simulink model "sofc_system5_mpc11_int"  (Simulink 7.6)
settings: Solver=FixedStepDiscrete  StartTime=0.0  StopTime=3500  FixedStep=1  MaxStep=1  RelTol=1e-3
settings Model: Creator=Ben  LastModifiedBy=Ben

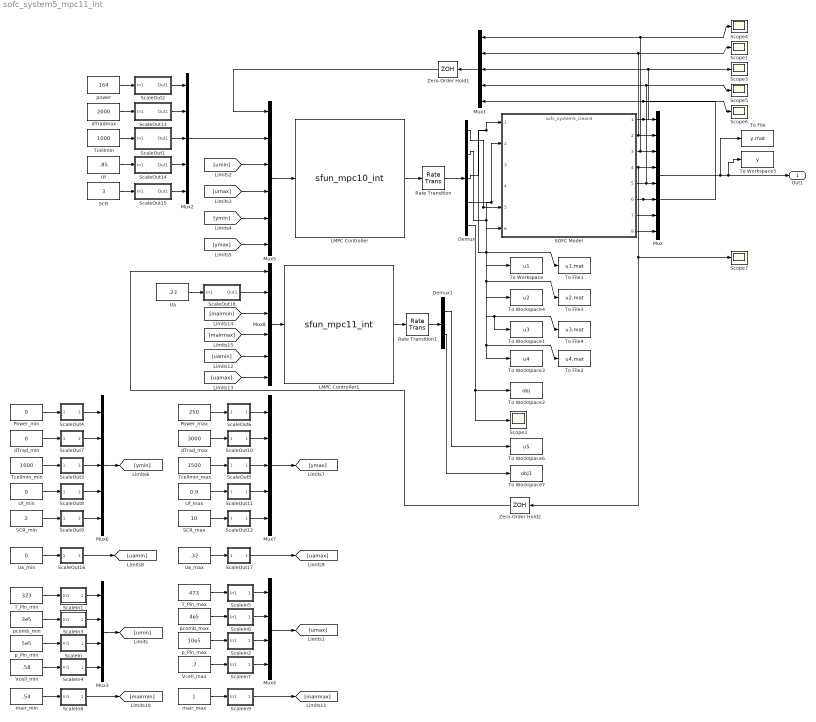
== system sofc_system5_mpc11_int ==
  Demux : Demux  Outputs=5
  Demux1 : Demux  Outputs=2
  LMPC Controller : S-Function  Priority=3  FunctionName=sfun_mpc10_int  EnableBusSupport=off
  LMPC Controller1 : S-Function  Priority=3  FunctionName=sfun_mpc11_int  EnableBusSupport=off
  Mux : Mux  Inputs=8
  Mux{1..2,6..7} (4 alike) : Mux  Inputs=5
  Mux3 : Mux
  Mux4 : Mux
  Mux5 : Mux  Inputs=6
  Mux8 : Mux  Inputs=6
  Power_max : Constant  Priority=1  Value=250
  Power_min : Constant  Priority=1  Value=0
  Rate Transition : RateTransition  Deterministic=off  OutPortSampleTimeMultiple=5  OutPortSampleTime=1
  Rate Transition1 : RateTransition  Deterministic=off  OutPortSampleTimeMultiple=5  OutPortSampleTime=1
  SCR : Constant  Priority=1  Value=3
  SCR_max : Constant  Priority=1  Value=10
  SCR_min : Constant  Priority=1  Value=2
  SOFC Model : ModelReference  Priority=1  ModelNameDialog=sofc_system5_clean3  SimulationMode=Normal  ModelReferenceVersion=1.62  CopyOfModelName=sofc_system5_clean3
      mask Display: image(imread('sofc.png'))
  ScaleIn : Subsystem
  ScaleIn1 : Subsystem
  ScaleIn2 : Subsystem
  ScaleIn3 : Subsystem
  ScaleIn4 : Subsystem
  ScaleIn5 : Subsystem
  ScaleIn6 : Subsystem
  ScaleIn7 : Subsystem
  ScaleIn8 : Subsystem
  ScaleIn9 : Subsystem
  ScaleOut1 : Subsystem  Priority=1
  ScaleOut10 : Subsystem  Priority=1
  ScaleOut11 : Subsystem  Priority=1
  ScaleOut12 : Subsystem  Priority=1
  ScaleOut13 : Subsystem  Priority=1
  ScaleOut14 : Subsystem  Priority=1
  ScaleOut15 : Subsystem  Priority=1
  ScaleOut16 : Subsystem  Priority=1
  ScaleOut17 : Subsystem  Priority=1
  ScaleOut18 : Subsystem  Priority=1
  ScaleOut2 : Subsystem  Priority=1
  ScaleOut3 : Subsystem  Priority=1
  ScaleOut4 : Subsystem  Priority=1
  ScaleOut5 : Subsystem  Priority=1
  ScaleOut6 : Subsystem  Priority=1
  ScaleOut7 : Subsystem  Priority=1
  ScaleOut8 : Subsystem  Priority=1
  ScaleOut9 : Subsystem  Priority=1
  Scope{1..7} (7 alike) : Scope
      Scope1 settings: YMin=-0.125  YMax=0.15
      Scope2 settings: TimeRange=43.34600760456274  YMin=1645  YMax=1670  SaveName=ScopeData2
      Scope3 settings: YMin=1.85446  YMax=2.04966
      Scope4 settings: YMin=1.4787  YMax=1.4799  SaveName=ScopeData4
      Scope5 settings: YMin=-0.125  YMax=0.15  SaveName=ScopeData3
      Scope6 settings: YMin=-0.125  YMax=0.15  SaveName=ScopeData5
      Scope7 settings: YMin=-0.125  YMax=0.15  SaveName=ScopeData6
  T_Pin_max : Constant  Priority=1  Value=473
  T_Pin_min : Constant  Priority=1  Value=323
  Tcellmin : Constant  Priority=1  Value=1000
  Tcellmin_max : Constant  Priority=1  Value=1500
  Tcellmin_min : Constant  Priority=1  Value=1000
  To File : ToFile  Filename=y.mat
  To File1 : ToFile  Filename=u1.mat
  To File2 : ToFile  Filename=u4.mat
  To File3 : ToFile  Filename=u2.mat
  To File4 : ToFile  Filename=u3.mat
  To Workspace : ToWorkspace  VariableName=u1  SampleTime=-1  SaveFormat=Structure
  To Workspace1 : ToWorkspace  VariableName=u3  SampleTime=-1  SaveFormat=Structure
  To Workspace2 : ToWorkspace  VariableName=obj  SampleTime=-1  SaveFormat=Structure
  To Workspace3 : ToWorkspace  VariableName=u4  SampleTime=-1  SaveFormat=Structure
  To Workspace4 : ToWorkspace  VariableName=u2  SampleTime=-1  SaveFormat=Structure
  To Workspace5 : ToWorkspace  VariableName=y  SampleTime=-1  SaveFormat=Structure
  To Workspace6 : ToWorkspace  VariableName=u5  SampleTime=-1  SaveFormat=Structure
  To Workspace7 : ToWorkspace  VariableName=obj1  SampleTime=-1  SaveFormat=Structure
  Ua : Constant  Priority=1  Value=.23
  Ua_max : Constant  Priority=1  Value=.32
  Ua_min : Constant  Priority=1  Value=0
  Uf : Constant  Priority=1  Value=.85
  Uf_max : Constant  Priority=1  Value=0.9
  Uf_min : Constant  Priority=1  Value=0
  Vcell_max : Constant  Priority=1  Value=.7
  Vcell_min : Constant  Priority=1  Value=.58
  Zero-Order Hold1 : ZeroOrderHold  SampleTime=10
  Zero-Order Hold2 : ZeroOrderHold  SampleTime=10
  dTrad_max : Constant  Priority=1  Value=3000
  dTrad_min : Constant  Priority=1  Value=0
  dTradmax : Constant  Priority=1  Value=2000
  mair_max : Constant  Priority=1
  mair_min : Constant  Priority=1  Value=.54
  p_Pin_max : Constant  Priority=1  Value=10e5
  p_Pin_min : Constant  Priority=1  Value=5e5
  pcomb_max : Constant  Priority=1  Value=4e5
  pcomb_min : Constant  Priority=1  Value=3e5
  power : Constant  Priority=1  Value=164
  Out1 : Outport
  wires:
  SOFC Model/1 -> Mux/1, Mux1/3, Scope3/1
  SOFC Model/2 -> Mux/2, Mux1/2, Scope1/1
  SOFC Model/3 -> Mux/3, Mux1/1, Scope4/1
  SOFC Model/4 -> Mux/4, Scope7/1, Zero-Order Hold2/1
  SOFC Model/5 -> Mux/5, Mux1/4, Scope5/1
  SOFC Model/6 -> Mux/6, Scope6/1, Mux1/5
  Mux/1 -> Out1/1, To Workspace5/1, To File/1
  p_Pin_min/1 -> ScaleIn/1(In1)
  [umin] -> Mux5/3
  [umax] -> Mux5/4
  Mux5/1 -> LMPC Controller/1
  Zero-Order Hold1/1 -> Mux5/1
  power/1 -> ScaleOut2/1(In1)
  ScaleOut2/1(Out1) -> Mux2/1
  Mux2/1 -> Mux5/2
  T_Pin_min/1 -> ScaleIn1/1(In1)
  Mux3/1 -> [umin]
  Mux1/1 -> Zero-Order Hold1/1
  [ymax] -> Mux5/6
  [ymin] -> Mux5/5
  Power_min/1 -> ScaleOut4/1(In1)
  Tcellmin_min/1 -> ScaleOut3/1(In1)
  Mux6/1 -> [ymin]
  ScaleOut4/1(Out1) -> Mux6/1
  SOFC Model/7 -> Mux/7
  SOFC Model/8 -> Mux/8
  LMPC Controller/1 -> Rate Transition/1
  Rate Transition/1 -> Demux/1
  Demux/5 -> Scope2/1, To Workspace2/1
  Tcellmin/1 -> ScaleOut1/1(In1)
  ScaleOut3/1(Out1) -> Mux6/3
  dTrad_min/1 -> ScaleOut7/1(In1)
  ScaleOut7/1(Out1) -> Mux6/2
  Uf_min/1 -> ScaleOut8/1(In1)
  ScaleOut8/1(Out1) -> Mux6/4
  SCR_min/1 -> ScaleOut9/1(In1)
  ScaleOut9/1(Out1) -> Mux6/5
  Power_max/1 -> ScaleOut6/1(In1)
  Tcellmin_max/1 -> ScaleOut5/1(In1)
  Mux7/1 -> [ymax]
  ScaleOut6/1(Out1) -> Mux7/1
  ScaleOut5/1(Out1) -> Mux7/3
  dTrad_max/1 -> ScaleOut10/1(In1)
  ScaleOut10/1(Out1) -> Mux7/2
  Uf_max/1 -> ScaleOut11/1(In1)
  ScaleOut11/1(Out1) -> Mux7/4
  SCR_max/1 -> ScaleOut12/1(In1)
  ScaleOut12/1(Out1) -> Mux7/5
  ScaleIn1/1(Out1) -> Mux3/1
  ScaleIn/1(Out1) -> Mux3/3
  pcomb_min/1 -> ScaleIn3/1(In1)
  ScaleIn3/1(Out1) -> Mux3/2
  Vcell_min/1 -> ScaleIn4/1(In1)
  ScaleIn4/1(Out1) -> Mux3/4
  p_Pin_max/1 -> ScaleIn2/1(In1)
  T_Pin_max/1 -> ScaleIn5/1(In1)
  Mux4/1 -> [umax]
  ScaleIn5/1(Out1) -> Mux4/1
  ScaleIn2/1(Out1) -> Mux4/3
  pcomb_max/1 -> ScaleIn6/1(In1)
  ScaleIn6/1(Out1) -> Mux4/2
  Vcell_max/1 -> ScaleIn7/1(In1)
  ScaleIn7/1(Out1) -> Mux4/4
  ScaleOut1/1(Out1) -> Mux2/3
  dTradmax/1 -> ScaleOut13/1(In1)
  ScaleOut13/1(Out1) -> Mux2/2
  Uf/1 -> ScaleOut14/1(In1)
  ScaleOut14/1(Out1) -> Mux2/4
  SCR/1 -> ScaleOut15/1(In1)
  ScaleOut15/1(Out1) -> Mux2/5
  Demux/3 -> SOFC Model/1, To Workspace/1, To File1/1
  Demux/4 -> SOFC Model/2, To Workspace4/1, To File3/1
  Demux/2 -> SOFC Model/6, To Workspace3/1, To File2/1
  Demux/1 -> SOFC Model/5, To Workspace1/1, To File4/1
  Ua_min/1 -> ScaleOut16/1(In1)
  ScaleOut16/1(Out1) -> [uamin]
  Ua_max/1 -> ScaleOut17/1(In1)
  ScaleOut17/1(Out1) -> [uamax]
  mair_min/1 -> ScaleIn8/1(In1)
  ScaleIn8/1(Out1) -> [mairmin]
  mair_max/1 -> ScaleIn9/1(In1)
  ScaleIn9/1(Out1) -> [mairmax]
  Ua/1 -> ScaleOut18/1(In1)
  ScaleOut18/1(Out1) -> Mux8/2
  [uamax] -> Mux8/6
  [uamin] -> Mux8/5
  [mairmax] -> Mux8/4
  [mairmin] -> Mux8/3
  Mux8/1 -> LMPC Controller1/1
  LMPC Controller1/1 -> Rate Transition1/1
  Zero-Order Hold2/1 -> Mux8/1
  Rate Transition1/1 -> Demux1/1
  Demux1/1 -> To Workspace6/1
  Demux1/2 -> To Workspace7/1

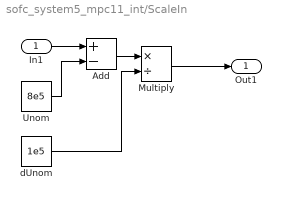
== system sofc_system5_mpc11_int/ScaleIn ==
  In1 : Inport
  Add : Sum  Inputs=+-
  Multiply : Product  Inputs=*/
  Unom : Constant  Value=8e5
  dUnom : Constant  Value=1e5
  Out1 : Outport
  wires:
  Unom/1 -> Add/2
  In1/1 -> Add/1
  Add/1 -> Multiply/1
  dUnom/1 -> Multiply/2
  Multiply/1 -> Out1/1

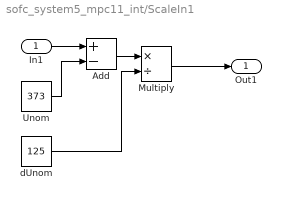
== system sofc_system5_mpc11_int/ScaleIn1 ==
  In1 : Inport
  Add : Sum  Inputs=+-
  Multiply : Product  Inputs=*/
  Unom : Constant  Value=373
  dUnom : Constant  Value=125
  Out1 : Outport
  wires:
  Unom/1 -> Add/2
  In1/1 -> Add/1
  Add/1 -> Multiply/1
  dUnom/1 -> Multiply/2
  Multiply/1 -> Out1/1

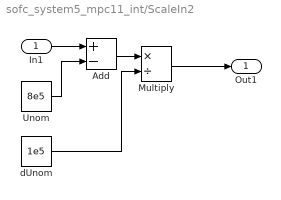
== system sofc_system5_mpc11_int/ScaleIn2 ==
  In1 : Inport
  Add : Sum  Inputs=+-
  Multiply : Product  Inputs=*/
  Unom : Constant  Value=8e5
  dUnom : Constant  Value=1e5
  Out1 : Outport
  wires:
  Unom/1 -> Add/2
  In1/1 -> Add/1
  Add/1 -> Multiply/1
  dUnom/1 -> Multiply/2
  Multiply/1 -> Out1/1

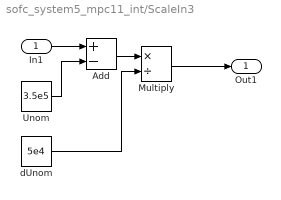
== system sofc_system5_mpc11_int/ScaleIn3 ==
  In1 : Inport
  Add : Sum  Inputs=+-
  Multiply : Product  Inputs=*/
  Unom : Constant  Value=3.5e5
  dUnom : Constant  Value=5e4
  Out1 : Outport
  wires:
  Unom/1 -> Add/2
  In1/1 -> Add/1
  Add/1 -> Multiply/1
  dUnom/1 -> Multiply/2
  Multiply/1 -> Out1/1

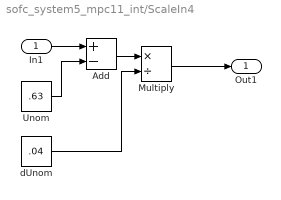
== system sofc_system5_mpc11_int/ScaleIn4 ==
  In1 : Inport
  Add : Sum  Inputs=+-
  Multiply : Product  Inputs=*/
  Unom : Constant  Value=.63
  dUnom : Constant  Value=.04
  Out1 : Outport
  wires:
  Unom/1 -> Add/2
  In1/1 -> Add/1
  Add/1 -> Multiply/1
  dUnom/1 -> Multiply/2
  Multiply/1 -> Out1/1

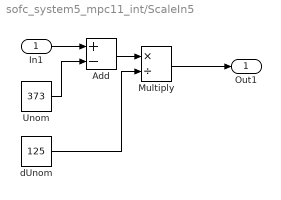
== system sofc_system5_mpc11_int/ScaleIn5 ==
  In1 : Inport
  Add : Sum  Inputs=+-
  Multiply : Product  Inputs=*/
  Unom : Constant  Value=373
  dUnom : Constant  Value=125
  Out1 : Outport
  wires:
  Unom/1 -> Add/2
  In1/1 -> Add/1
  Add/1 -> Multiply/1
  dUnom/1 -> Multiply/2
  Multiply/1 -> Out1/1

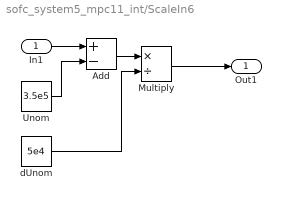
== system sofc_system5_mpc11_int/ScaleIn6 ==
  In1 : Inport
  Add : Sum  Inputs=+-
  Multiply : Product  Inputs=*/
  Unom : Constant  Value=3.5e5
  dUnom : Constant  Value=5e4
  Out1 : Outport
  wires:
  Unom/1 -> Add/2
  In1/1 -> Add/1
  Add/1 -> Multiply/1
  dUnom/1 -> Multiply/2
  Multiply/1 -> Out1/1

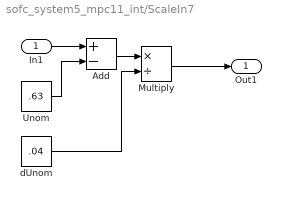
== system sofc_system5_mpc11_int/ScaleIn7 ==
  In1 : Inport
  Add : Sum  Inputs=+-
  Multiply : Product  Inputs=*/
  Unom : Constant  Value=.63
  dUnom : Constant  Value=.04
  Out1 : Outport
  wires:
  Unom/1 -> Add/2
  In1/1 -> Add/1
  Add/1 -> Multiply/1
  dUnom/1 -> Multiply/2
  Multiply/1 -> Out1/1

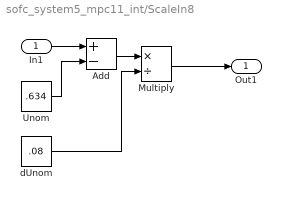
== system sofc_system5_mpc11_int/ScaleIn8 ==
  In1 : Inport
  Add : Sum  Inputs=+-
  Multiply : Product  Inputs=*/
  Unom : Constant  Value=.634
  dUnom : Constant  Value=.08
  Out1 : Outport
  wires:
  Unom/1 -> Add/2
  In1/1 -> Add/1
  Add/1 -> Multiply/1
  dUnom/1 -> Multiply/2
  Multiply/1 -> Out1/1

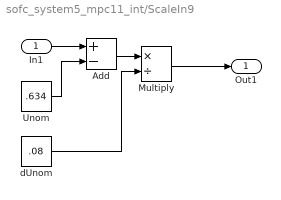
== system sofc_system5_mpc11_int/ScaleIn9 ==
  In1 : Inport
  Add : Sum  Inputs=+-
  Multiply : Product  Inputs=*/
  Unom : Constant  Value=.634
  dUnom : Constant  Value=.08
  Out1 : Outport
  wires:
  Unom/1 -> Add/2
  In1/1 -> Add/1
  Add/1 -> Multiply/1
  dUnom/1 -> Multiply/2
  Multiply/1 -> Out1/1

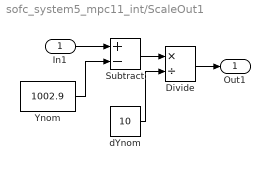
== system sofc_system5_mpc11_int/ScaleOut1 ==
  In1 : Inport
  Divide : Product  Inputs=*/
  Subtract : Sum  Inputs=+-
  Ynom : Constant  Value=1002.9
  dYnom : Constant  Value=10
  Out1 : Outport
  wires:
  In1/1 -> Subtract/1
  Ynom/1 -> Subtract/2
  Subtract/1 -> Divide/1
  Divide/1 -> Out1/1
  dYnom/1 -> Divide/2

== system sofc_system5_mpc11_int/ScaleOut10 ==
  In1 : Inport
  Divide : Product  Inputs=*/
  Subtract : Sum  Inputs=+-
  Ynom : Constant  Value=2337.6
  dYnom : Constant  Value=350
  Out1 : Outport
  wires:
  In1/1 -> Subtract/1
  Ynom/1 -> Subtract/2
  Subtract/1 -> Divide/1
  Divide/1 -> Out1/1
  dYnom/1 -> Divide/2

== system sofc_system5_mpc11_int/ScaleOut11 ==
  In1 : Inport
  Divide : Product  Inputs=*/
  Subtract : Sum  Inputs=+-
  Ynom : Constant  Value=.7434
  dYnom : Constant  Value=.1
  Out1 : Outport
  wires:
  In1/1 -> Subtract/1
  Ynom/1 -> Subtract/2
  Subtract/1 -> Divide/1
  Divide/1 -> Out1/1
  dYnom/1 -> Divide/2

== system sofc_system5_mpc11_int/ScaleOut12 ==
  In1 : Inport
  Divide : Product  Inputs=*/
  Subtract : Sum  Inputs=+-
  Ynom : Constant  Value=2.2325
  dYnom : Constant  Value=1.2
  Out1 : Outport
  wires:
  In1/1 -> Subtract/1
  Ynom/1 -> Subtract/2
  Subtract/1 -> Divide/1
  Divide/1 -> Out1/1
  dYnom/1 -> Divide/2

== system sofc_system5_mpc11_int/ScaleOut13 ==
  In1 : Inport
  Divide : Product  Inputs=*/
  Subtract : Sum  Inputs=+-
  Ynom : Constant  Value=2337.6
  dYnom : Constant  Value=350
  Out1 : Outport
  wires:
  In1/1 -> Subtract/1
  Ynom/1 -> Subtract/2
  Subtract/1 -> Divide/1
  Divide/1 -> Out1/1
  dYnom/1 -> Divide/2

== system sofc_system5_mpc11_int/ScaleOut14 ==
  In1 : Inport
  Divide : Product  Inputs=*/
  Subtract : Sum  Inputs=+-
  Ynom : Constant  Value=.7434
  dYnom : Constant  Value=.1
  Out1 : Outport
  wires:
  In1/1 -> Subtract/1
  Ynom/1 -> Subtract/2
  Subtract/1 -> Divide/1
  Divide/1 -> Out1/1
  dYnom/1 -> Divide/2

== system sofc_system5_mpc11_int/ScaleOut15 ==
  In1 : Inport
  Divide : Product  Inputs=*/
  Subtract : Sum  Inputs=+-
  Ynom : Constant  Value=2.2325
  dYnom : Constant  Value=1.2
  Out1 : Outport
  wires:
  In1/1 -> Subtract/1
  Ynom/1 -> Subtract/2
  Subtract/1 -> Divide/1
  Divide/1 -> Out1/1
  dYnom/1 -> Divide/2

== system sofc_system5_mpc11_int/ScaleOut16 ==
  In1 : Inport
  Divide : Product  Inputs=*/
  Subtract : Sum  Inputs=+-
  Ynom : Constant  Value=.23151
  dYnom : Constant  Value=.015
  Out1 : Outport
  wires:
  In1/1 -> Subtract/1
  Ynom/1 -> Subtract/2
  Subtract/1 -> Divide/1
  Divide/1 -> Out1/1
  dYnom/1 -> Divide/2

== system sofc_system5_mpc11_int/ScaleOut17 ==
  In1 : Inport
  Divide : Product  Inputs=*/
  Subtract : Sum  Inputs=+-
  Ynom : Constant  Value=.23151
  dYnom : Constant  Value=.015
  Out1 : Outport
  wires:
  In1/1 -> Subtract/1
  Ynom/1 -> Subtract/2
  Subtract/1 -> Divide/1
  Divide/1 -> Out1/1
  dYnom/1 -> Divide/2

== system sofc_system5_mpc11_int/ScaleOut18 ==
  In1 : Inport
  Divide : Product  Inputs=*/
  Subtract : Sum  Inputs=+-
  Ynom : Constant  Value=.23151
  dYnom : Constant  Value=.015
  Out1 : Outport
  wires:
  In1/1 -> Subtract/1
  Ynom/1 -> Subtract/2
  Subtract/1 -> Divide/1
  Divide/1 -> Out1/1
  dYnom/1 -> Divide/2

== system sofc_system5_mpc11_int/ScaleOut2 ==
  In1 : Inport
  Divide : Product  Inputs=*/
  Subtract : Sum  Inputs=+-
  Ynom : Constant  Value=153.52
  dYnom : Constant  Value=8
  Out1 : Outport
  wires:
  In1/1 -> Subtract/1
  Ynom/1 -> Subtract/2
  Subtract/1 -> Divide/1
  Divide/1 -> Out1/1
  dYnom/1 -> Divide/2

== system sofc_system5_mpc11_int/ScaleOut3 ==
  In1 : Inport
  Divide : Product  Inputs=*/
  Subtract : Sum  Inputs=+-
  Ynom : Constant  Value=1002.9
  dYnom : Constant  Value=10
  Out1 : Outport
  wires:
  In1/1 -> Subtract/1
  Ynom/1 -> Subtract/2
  Subtract/1 -> Divide/1
  Divide/1 -> Out1/1
  dYnom/1 -> Divide/2

== system sofc_system5_mpc11_int/ScaleOut4 ==
  In1 : Inport
  Divide : Product  Inputs=*/
  Subtract : Sum  Inputs=+-
  Ynom : Constant  Value=153.52
  dYnom : Constant  Value=8
  Out1 : Outport
  wires:
  In1/1 -> Subtract/1
  Ynom/1 -> Subtract/2
  Subtract/1 -> Divide/1
  Divide/1 -> Out1/1
  dYnom/1 -> Divide/2

== system sofc_system5_mpc11_int/ScaleOut5 ==
  In1 : Inport
  Divide : Product  Inputs=*/
  Subtract : Sum  Inputs=+-
  Ynom : Constant  Value=1002.9
  dYnom : Constant  Value=10
  Out1 : Outport
  wires:
  In1/1 -> Subtract/1
  Ynom/1 -> Subtract/2
  Subtract/1 -> Divide/1
  Divide/1 -> Out1/1
  dYnom/1 -> Divide/2

== system sofc_system5_mpc11_int/ScaleOut6 ==
  In1 : Inport
  Divide : Product  Inputs=*/
  Subtract : Sum  Inputs=+-
  Ynom : Constant  Value=153.52
  dYnom : Constant  Value=8
  Out1 : Outport
  wires:
  In1/1 -> Subtract/1
  Ynom/1 -> Subtract/2
  Subtract/1 -> Divide/1
  Divide/1 -> Out1/1
  dYnom/1 -> Divide/2

== system sofc_system5_mpc11_int/ScaleOut7 ==
  In1 : Inport
  Divide : Product  Inputs=*/
  Subtract : Sum  Inputs=+-
  Ynom : Constant  Value=2337.6
  dYnom : Constant  Value=350
  Out1 : Outport
  wires:
  In1/1 -> Subtract/1
  Ynom/1 -> Subtract/2
  Subtract/1 -> Divide/1
  Divide/1 -> Out1/1
  dYnom/1 -> Divide/2

== system sofc_system5_mpc11_int/ScaleOut8 ==
  In1 : Inport
  Divide : Product  Inputs=*/
  Subtract : Sum  Inputs=+-
  Ynom : Constant  Value=.7434
  dYnom : Constant  Value=.1
  Out1 : Outport
  wires:
  In1/1 -> Subtract/1
  Ynom/1 -> Subtract/2
  Subtract/1 -> Divide/1
  Divide/1 -> Out1/1
  dYnom/1 -> Divide/2

== system sofc_system5_mpc11_int/ScaleOut9 ==
  In1 : Inport
  Divide : Product  Inputs=*/
  Subtract : Sum  Inputs=+-
  Ynom : Constant  Value=2.2325
  dYnom : Constant  Value=1.2
  Out1 : Outport
  wires:
  In1/1 -> Subtract/1
  Ynom/1 -> Subtract/2
  Subtract/1 -> Divide/1
  Divide/1 -> Out1/1
  dYnom/1 -> Divide/2
